simulink model "bpsk"  (Simulink 6.4)
settings: Solver=FixedStepDiscrete  StartTime=0.0  StopTime=inf  RelTol=1e-3
libraries: commdigbbndpm3 x2, commsink2 x2, commchan3 x1, commrandsrc2 x1
settings Model: Creator=ALEX  LastModifiedBy=student
settings OptimizationCC: InitFltsAndDblsToZero=off
settings DebuggingCC: SignalResolutionControl=UseLocalSettings  MultiTaskDSMMsg=error  MultiTaskCondExecSysMsg=error
settings GRTTargetCC: TargetFcnLib=ansi_tfl_table_tmw.mat

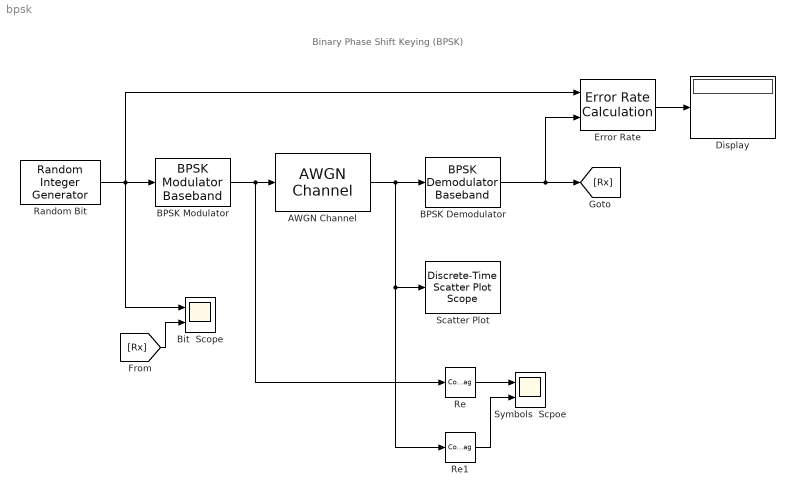
== system bpsk ==
  note: Binary Phase Shift Keying (BPSK)
  AWGN Channel : commchan3/AWGN Channel  SystemSampleTime=-1  seed=33  noiseMode="Signal to noise ratio  (Es/No)"  EbNodB=3  EsNodB=100  SNRdB=10  bitsPerSym=1  Ps=1  Tsym=1  variance=0.2
  BPSK Demodulator : commdigbbndpm3/BPSK Demodulator Baseband  SystemSampleTime=-1  Ph=0  outDtype=boolean
  BPSK Modulator : commdigbbndpm3/BPSK Modulator Baseband  SystemSampleTime=-1  Ph=0  outDtype=double  outWordLen=16  outUDDataType=sfix(16)  outFracLenMode=Best precision  outFracLen=15
  "Bit  Scope " : Scope  NumInputPorts=2
      settings: YMin=0~0  YMax=1.2~1.2
  Display : Display
  Error Rate : commsink2/Error Rate Calculation  N=0  st_delay=0  cp_mode=Entire frame  subframe=[]  PMode=Port  WsName=ErrorVec  RsMode2=off  stop=off  numErr=10000  maxBits=100000
  Random Bit : commrandsrc2/Random Integer Generator  SystemSampleTime=-1  mul=2  seed=63  Ts=1  frameBased=off  sampPerFrame=8  orient=off  outDataType=boolean
  Re : ComplexToRealImag  Output=Real
  Re1 : ComplexToRealImag  Output=Real
  Scatter Plot : commsink2/Discrete-Time Scatter Plot Scope  Tag=ScatterPlot  SystemSampleTime=-1  sampPerSymb=1  offsetEye=0  numTraces=100  numNewFrames=10  LineMarkers=.  LineColors=b  fading=on  render=on  AxisGrid=on  xMin=-2  xMax=2  yMin=-2  yMax=2  inphaseLabel=In-phase Amplitude  quadratureLabel=Quadrature Amplitude  openScopeAtSimStart=off  FrameNumber=off  FigPos=[360 362 560 560]  figTitle=Scatter Plot  numLinesMax=8  block_type_=scatter
  Symbols  Scpoe : Scope  NumInputPorts=2
      settings: TimeRange=20  YMin=-1.2~-2  YMax=1.2~2.5
  wires:
  AWGN Channel/1 -> BPSK Demodulator/1, Scatter Plot/1, Re1/1
  BPSK Demodulator/1 -> Error Rate/2, [Rx]
  Error Rate/1 -> Display/1
  Random Bit/1 -> BPSK Modulator/1, Error Rate/1, "Bit  Scope "/1
  BPSK Modulator/1 -> AWGN Channel/1, Re/1
  [Rx] -> "Bit  Scope "/2
  Re/1 -> Symbols  Scpoe/1
  Re1/1 -> Symbols  Scpoe/2
